simulink model "sensorExpoler1_4"  (R2026a)
settings: Solver=FixedStepAuto  StopTime=inf  FixedStep=0.001
undefined symbols (not defined in the file): Blocking, Non
libraries: amg_usbconverter_n_connect_lib x2
settings Model: Creator=pboon  LastModifiedBy=Itthiphat

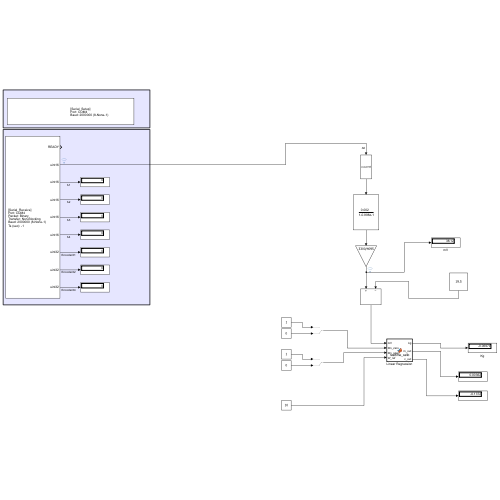
[thumbnail: Simulink's stored preview of the top-level diagram]
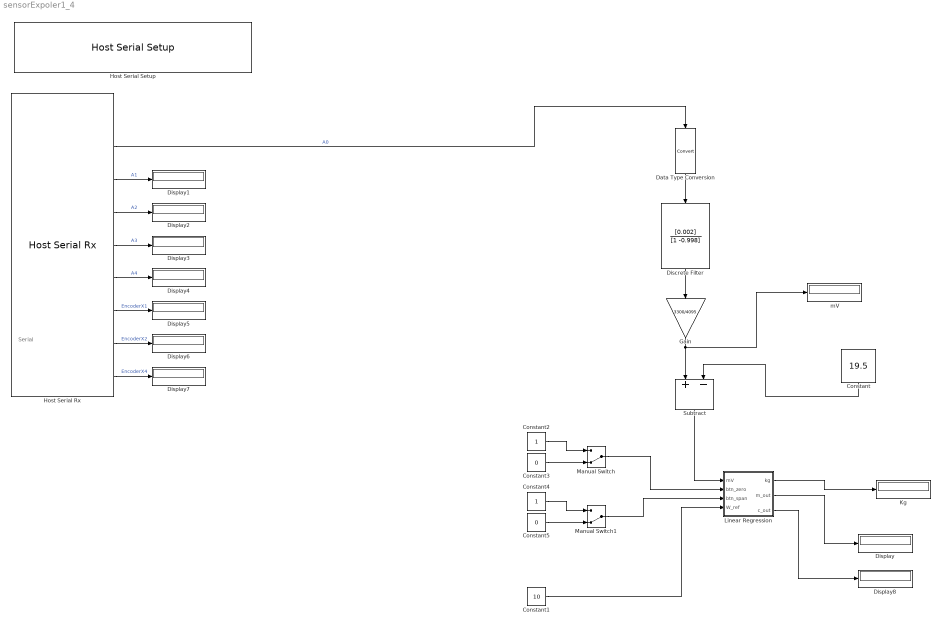
== system sensorExpoler1_4 ==
  note: Serial
  Constant : Constant  Value=19.5
  Constant1 : Constant  Value=10
  Constant2 : Constant
  Constant3 : Constant  Value=0
  Constant4 : Constant
  Constant5 : Constant  Value=0
  Data Type Conversion : DataTypeConversion  SaturateOnIntegerOverflow=off  RndMeth=Floor
  Discrete Filter : DiscreteFilter  Numerator=[0.002]  Denominator=[1 -0.998]
  Display{,1..8} (9 alike) : Display
  Gain : Gain  Gain=3300/4095
  Host Serial Rx : amg_usbconverter_n_connect_lib/Host Serial Rx  conf=rx  port=<auto>  baudrate=2000000  databits=8  parity=None  stopbit=1  flowcontrol=None  transfer=Non-Blocking  timeout=5  packetmode=Binary  enableinitialvalues=off  initialvalues=[]  binheader='25'  binterminator='4E 4E'  porttype_double=0  porttype_single=0  porttype_int8=0  porttype_uint8=0  porttype_int16=0  porttype_uint16=5  porttype_int32=0  porttype_uint32=3  asciiformat='%d,%f'  rx_asciiterminator="CRLF (0x0D 0x0A - \"\\r\\n\")"  tx_asciiterminator="CRLF (0x0D 0x0A - \"\\r\\n\")"  sampletime=0.001  enablecustomportlabel=off  cinputportlabel=0  coutputportlabel=A  portpinstr=0  blockid=HostSerialRx  inputporttype=[]  inputportwidth=[]  inputportlabel={}  outputporttype=[3 5 5 5 5 5 7 7 7]  outputportwidth=[1 1 1 1 1 1 1 1 1]  outputportlabel={'READY','uint16','uint16','uint16','uint16','uint16','uint32','uint32','uint32'}  compat=0  optionstring=[]  autoport='COM4'
  Host Serial Setup : amg_usbconverter_n_connect_lib/Host Serial Setup  conf=setup  port=<auto>  baudrate=2000000  databits=8  parity=None  stopbit=1  flowcontrol=None  transfer=Blocking  timeout=2  packetmode=Binary  initialvalues=[]  binheader='7E 7E'  binterminator='03 03'  porttype_double=0  porttype_single=1  porttype_int8=0  porttype_uint8=0  porttype_int16=0  porttype_uint16=0  porttype_int32=0  porttype_uint32=2  asciiformat='%d %u %x'  rx_asciiterminator="CRLF (0x0D 0x0A - \"\\r\\n\")"  tx_asciiterminator="CRLF (0x0D 0x0A - \"\\r\\n\")"  sampletime=-1  enablecustomportlabel=off  cinputportlabel=0  coutputportlabel=A  portpinstr=0  blockid=HostSerialSetup  inputporttype=[]  inputportwidth=[]  inputportlabel={}  outputporttype=[]  outputportwidth=[]  outputportlabel={}  compat=0  optionstring=[]  autoport='COM4'
  Kg : Display
  Linear Regression : MATLAB Function  TreatAsAtomicUnit=on
  Manual Switch : ManualSwitch  CurrentSetting=0
  Manual Switch1 : ManualSwitch  CurrentSetting=0
  Subtract : Sum  Inputs=+-
  mV : Display
  wires:
  Host Serial Rx/2 -> Data Type Conversion/1  "A0"
  Host Serial Rx/3 -> Display1/1  "A1"
  Host Serial Rx/4 -> Display2/1  "A2"
  Host Serial Rx/5 -> Display3/1  "A3"
  Host Serial Rx/6 -> Display4/1  "A4"
  Host Serial Rx/7 -> Display5/1  "EncoderX1"
  Host Serial Rx/8 -> Display6/1  "EncoderX2"
  Host Serial Rx/9 -> Display7/1  "EncoderX4"
  Data Type Conversion/1 -> Discrete Filter/1
  Discrete Filter/1 -> Gain/1
  Gain/1 -> mV/1, Subtract/1
  Constant/1 -> Subtract/2
  Linear Regression/1(kg) -> Kg/1
  Subtract/1 -> Linear Regression/1(mV)
  Constant1/1 -> Linear Regression/4(W_ref)
  Constant2/1 -> Manual Switch/1
  Constant3/1 -> Manual Switch/2
  Manual Switch/1 -> Linear Regression/2(btn_zero)
  Constant4/1 -> Manual Switch1/1
  Constant5/1 -> Manual Switch1/2
  Manual Switch1/1 -> Linear Regression/3(btn_span)
  Linear Regression/2(m_out) -> Display/1
  Linear Regression/3(c_out) -> Display8/1

== matlab function sensorExpoler1_4/Linear Regression ==
  data: mV input; kg output; btn_zero input; btn_span input; W_ref input; m_out output; c_out output
function [kg, m_out, c_out] = realtime_calib(mV, btn_zero, btn_span, W_ref)
    % ใช้ persistent บันทึกค่าความจำข้าม Step
    persistent V_zero V_span m c last_btn_zero last_btn_span
    
    % กำหนดค่าเริ่มต้นครั้งแรกเมื่อเริ่มรัน Simulation
    if isempty(V_zero)
        V_zero = 37.9;         % ค่าแรงดัน Offset เริ่มต้นที่ 0 kg (mV)
        V_span = 2800.0;       % ค่าแรงดันคาดการณ์ที่ 10 kg (mV)
        m = 10.0 / (V_span - V_zero);
        c = -m * V_zero;
        last_btn_zero = 0;
        last_btn_span = 0;
    end

    % ตรวจจับสัญญาณขาขึ้น (0 -> 1) ของปุ่ม Tare (0 kg)
    if (btn_zero > 0.5) && (last_btn_zero <= 0.5)
        V_zero = mV;
        if abs(V_span - V_zero) > 0.001
            m = W_ref / (V_span - V_zero);
            c = -m * V_zero;
        end
    end

    % ตรวจจับสัญญาณขาขึ้น (0 -> 1) ของปุ่ม Calib (10 kg)
    if (btn_span > 0.5) && (last_btn_span <= 0.5)
        V_span = mV;
        if abs(V_span - V_zero) > 0.001
            m = W_ref / (V_span - V_zero);
            c = -m * V_zero;
        end
    end

    % บันทึกสถานะปุ่มกดปัจจุบันไว้เปรียบเทียบใน Step ถัดไป
    last_btn_zero = btn_zero;
    last_btn_span = btn_span;

    % คำนวณสมการเส้นตรง y = mx + c
    kg = m * mV + c;
    m_out = m;
    c_out = c;
end
